simulink model "ev_project_1"  (R2024b)
settings: Solver=VariableStepAuto  StartTime=0.0  StopTime=20  RelTol=1e-3
libraries: spsIGBTDiodeLib x12, spsDiodeLib x6, spsSeriesRLCBranchLib x3, spsVoltageMeasurementLib x3, spsDCVoltageSourceLib x1, spsGroundLib x1, spsPermanentMagnetSynchronousMachineLib x1, spsThreePhaseVIMeasurementLib x1, sps_lib x1
settings Model: Creator=ravit  LastModifiedBy=ravit

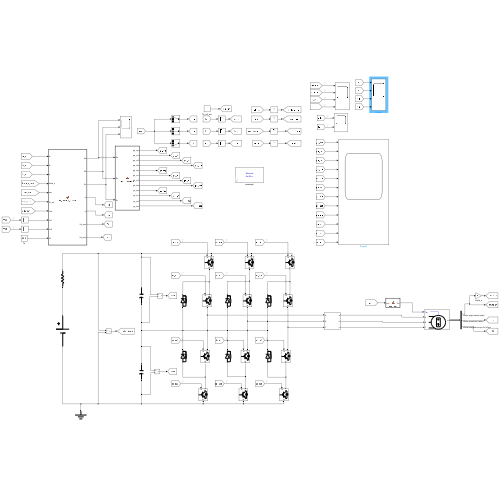
[thumbnail: Simulink's stored preview of the top-level diagram]
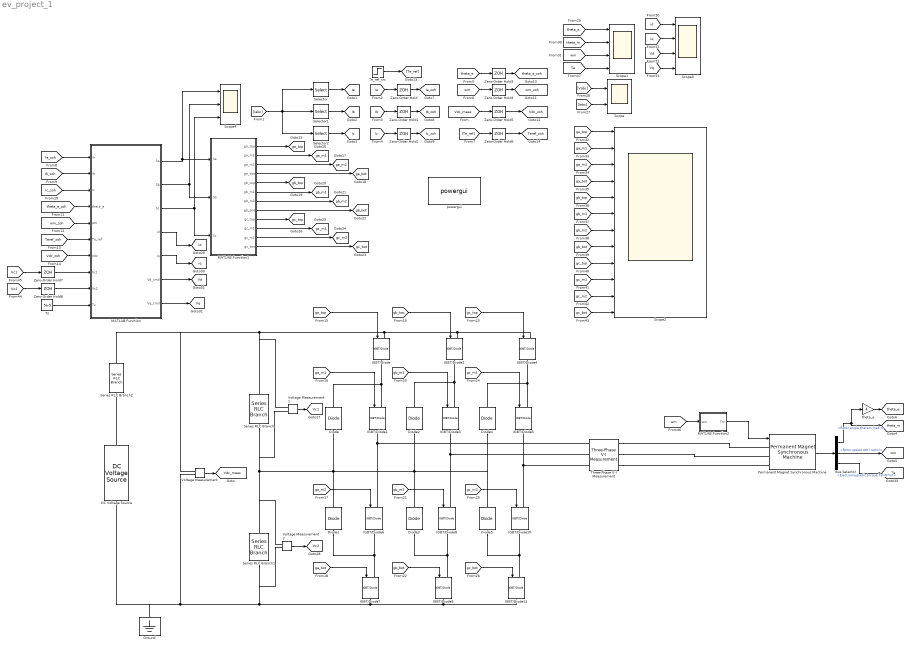
== system ev_project_1 ==
  Bus Selector : BusSelector  OutputSignals=Rotor angle thetam (rad),Rotor speed wm (rad/s),Electromagnetic torque Te (N*m)
  DC Voltage Source : spsDCVoltageSourceLib/DC Voltage Source  Amplitude=400  Measurements=None
  Diode{,1..5} (6 alike) : spsDiodeLib/Diode  Ron=0.001  Lon=0  Vf=0.8  IC=0  UseSnubber=0  Rs=500  Cs=250e-9  Measurements=off
  Ground : spsGroundLib/Ground  LConnTagsString=a
  IGBT/Diode{,1..11} (12 alike) : spsIGBTDiodeLib/IGBT//Diode  Ron=1e-3  Rs=1e5  Cs=inf  Measurements=off
  MATLAB Function : MATLAB Function  TreatAsAtomicUnit=on
  MATLAB Function1 : MATLAB Function  TreatAsAtomicUnit=on
  MATLAB Function2 : MATLAB Function  TreatAsAtomicUnit=on
  Permanent Magnet Synchronous Machine : spsPermanentMagnetSynchronousMachineLib/Permanent Magnet Synchronous Machine  NbPhases=3  FluxDistribution=Sinusoidal  RotorType=Salient-pole  MechanicalLoad=Torque Tm  PresetModel=No  ShowDetailedParameters=on  MeasurementBus=off  Resistance=0.05  Inductance=8.5e-3  dqInductances=[0.0005, 0.0011]  La=0.000395  MachineConstant=Flux linkage established by magnets (V.s)  Flux=0.045  VoltageCst=32.6484  TorqueCst=0.27  Flat=120  Mechanical=[0.01, 0.0004924, 4, 0]  PolePairs=4  InitialConditions=[0,0, 0,0]  InitialConditions5ph=[0 0 0 0 0 0]  RefAngle=90 degrees behind phase A axis (modified Park)  IterativeDiscreteModel=Trapezoidal non iterative  TsBlock=-1  TsPowergui=0
  Scope : Scope  NumInputPorts=2
  Scope1 : Scope  NumInputPorts=4
  Scope2 : Scope  NumInputPorts=12
  Scope3 : Scope  NumInputPorts=4
  Scope4 : Scope  NumInputPorts=3
  Selector : Selector  InputPortWidth=3  IndexOptions=Index vector (dialog)  Indices=[1]  OutputSizes=1
  Selector1 : Selector  InputPortWidth=3  IndexOptions=Index vector (dialog)  Indices=[2]  OutputSizes=1
  Selector2 : Selector  InputPortWidth=3  IndexOptions=Index vector (dialog)  Indices=[3]  OutputSizes=1
  Series RLC Branch : spsSeriesRLCBranchLib/Series RLC Branch  LConnTagsString=__new0  RConnTagsString=__new0  BranchType=C  Resistance=1  Inductance=1e-3  SetiL0=off  InitialCurrent=0  Capacitance=2200e-6  Setx0=on  InitialVoltage=200  Measurements=None
  Series RLC Branch1 : spsSeriesRLCBranchLib/Series RLC Branch  LConnTagsString=__new0  RConnTagsString=__new0  BranchType=C  Resistance=1  Inductance=1e-3  SetiL0=off  InitialCurrent=0  Capacitance=2200e-6  Setx0=on  InitialVoltage=200  Measurements=None
  Series RLC Branch2 : spsSeriesRLCBranchLib/Series RLC Branch  LConnTagsString=__new0  RConnTagsString=__new0  BranchType=R  Resistance=0.01  Inductance=1e-3  SetiL0=off  InitialCurrent=0  Capacitance=1e-6  Setx0=off  InitialVoltage=0  Measurements=None
  Te_ref_src : Step  Time=5  After=20  SampleTime=0
  Three-Phase V-I Measurement : spsThreePhaseVIMeasurementLib/Three-Phase V-I Measurement  VoltageMeasurement=phase-to-ground  SetLabelV=on  LabelV=Vabc  Vpu=off  VpuLL=off  CurrentMeasurement=yes  SetLabelI=on  LabelI=Iabc  Ipu=off  Pbase=100e6  Vbase=500e3  OutputType=Complex  PhasorSimulation=off  PSBequivalent=0
  Ts : Constant  Value=5e-5
  Voltage Measurement : spsVoltageMeasurementLib/Voltage Measurement  PhasorSimulation=off  OutputType=Complex  PSBequivalent=0
  Voltage Measurement1 : spsVoltageMeasurementLib/Voltage Measurement  PhasorSimulation=off  OutputType=Complex  PSBequivalent=0
  Voltage Measurement2 : spsVoltageMeasurementLib/Voltage Measurement  PhasorSimulation=off  OutputType=Complex  PSBequivalent=0
  Zero-Order Hold{,1..8} (9 alike) : ZeroOrderHold  SampleTime=5e-5
  powergui : sps_lib/powergui  Priority=1  SimulationMode=Discrete  SampleTime=50e-6  frequency=60  Iterations=50  frequencyindice=0  Pbase=100e6  ErrMax=1e-4  UnitsV=kV  UnitsW=MW  buscounter=0  FunctionMessages=off  echomessages=off  EnableUseOfTLC=off  CurrentSourceSwitches=off  DisableSnubberDevices=off  DisableRonSwitches=off  DisableVfSwitches=off  DisplayEquations=off  AutomaticDiscreteSolvers=off  SolverType=Tustin/Backward Euler (TBE)  Interpol=off  ExternalGateDelay=off  methode=off  Ts=100  x0status=blocks  SPID=on  SwTol=0  HookPort=off  NonlinearTolerance=1e-4  nMaxIteration=100  ContinueOnMaxIteration=off  RestoreLinks=warning  ResistiveCurrentMeasurement=off  Frange=[0:2:500]  Ylog=off  Xlog=on  ShowGrid=off  save=off  variable=ZData  structure=0  ZoomFFT=off  StartTime=0.0  cycles=1  DisplayStyle=1  fundamental=60  FreqAxis=off  MaxFrequency=1000  frequencyindicesteady=1  RmsSteady=1  display=off
  theta_e : Gain  Gain=4
  tag scope: Ia=global, Ia_zoh=global, Ib=global, Ib_zoh=global, Ic=global, Ic_zoh=global, Te=global, Teref_zoh=global, Vc1=global, Vc2=global, Vd=global, Vdc_meas=global, Vdc_zoh=global, Vq=global, ga_bot=global, ga_m1=global, ga_m2=global, ga_top=global, gb_bot=global, gb_m1=global, gb_m2=global, gb_top=global, gc_bot=global, gc_m1=global, gc_m2=global, gc_top=global, id=global, iq=global, theta_e=global, theta_e_zoh=global, theta_m=global, wm=global, wm_zoh=global
  wires:
  Voltage Measurement/1 -> [Vdc_meas]
  Permanent Magnet Synchronous Machine/1 -> Bus Selector/1
  [Iabc] -> Selector2/1, Selector/1, Selector1/1
  Selector/1 -> [Ia]
  Selector1/1 -> [Ib]
  Selector2/1 -> [Ic]
  Bus Selector/1 -> [theta_m], theta_e/1  "<Rotor angle thetam (rad)>"
  Bus Selector/2 -> [wm]  "<Rotor speed wm (rad/s)>"
  theta_e/1 -> [theta_e]
  [Ia] -> Zero-Order Hold/1
  [Ib] -> Zero-Order Hold1/1
  [Ic] -> Zero-Order Hold2/1
  Zero-Order Hold/1 -> [Ia_zoh]
  Zero-Order Hold1/1 -> [Ib_zoh]
  Zero-Order Hold2/1 -> [Ic_zoh]
  [theta_e] -> Zero-Order Hold3/1
  Zero-Order Hold3/1 -> [theta_e_zoh]
  [wm] -> Zero-Order Hold4/1
  Zero-Order Hold4/1 -> [wm_zoh]
  [Vdc_meas] -> Zero-Order Hold5/1
  Zero-Order Hold5/1 -> [Vdc_zoh]
  Te_ref_src/1 -> [Te_ref]
  [Te_ref] -> Zero-Order Hold6/1
  Zero-Order Hold6/1 -> [Teref_zoh]
  [Ia_zoh] -> MATLAB Function/1(ia)
  [Ib_zoh] -> MATLAB Function/2(ib)
  [Ic_zoh] -> MATLAB Function/3(ic)
  [theta_e_zoh] -> MATLAB Function/4(theta_e)
  [wm_zoh] -> MATLAB Function/5(wm)
  [Teref_zoh] -> MATLAB Function/6(Te_ref)
  [Vdc_zoh] -> MATLAB Function/7(Vdc)
  Ts/1 -> MATLAB Function/10(Ts)
  MATLAB Function/1(Sa) -> Scope4/1, MATLAB Function1/1(Sa)
  MATLAB Function/2(Sb) -> MATLAB Function1/2(Sb), Scope4/2
  MATLAB Function/3(Sc) -> MATLAB Function1/3(Sc), Scope4/3
  MATLAB Function1/1(ga_top) -> [ga_top]
  MATLAB Function1/2(ga_m1) -> [ga_m1]
  MATLAB Function1/3(ga_m2) -> [ga_m2]
  MATLAB Function1/4(ga_bot) -> [ga_bot]
  MATLAB Function1/5(gb_top) -> [gb_top]
  MATLAB Function1/6(gb_m1) -> [gb_m1]
  MATLAB Function1/7(gb_m2) -> [gb_m2]
  MATLAB Function1/8(gb_bot) -> [gb_bot]
  MATLAB Function1/12(gc_bot) -> [gc_bot]
  MATLAB Function1/11(gc_m2) -> [gc_m2]
  MATLAB Function1/10(gc_m1) -> [gc_m1]
  MATLAB Function1/9(gc_top) -> [gc_top]
  [ga_top] -> IGBT/Diode/1
  [ga_m1] -> IGBT/Diode1/1
  [ga_m2] -> IGBT/Diode6/1
  [ga_bot] -> IGBT/Diode7/1
  [gb_top] -> IGBT/Diode2/1
  [gb_m1] -> IGBT/Diode3/1
  [gb_m2] -> IGBT/Diode8/1
  [gb_bot] -> IGBT/Diode9/1
  [gc_top] -> IGBT/Diode4/1
  [gc_m2] -> IGBT/Diode10/1
  [gc_m1] -> IGBT/Diode5/1
  [gc_bot] -> IGBT/Diode11/1
  [Iabc] -> Scope/2
  [Vabc] -> Scope/1
  [theta_e] -> Scope1/1
  [theta_m] -> Scope1/2
  [wm] -> Scope1/3
  [ga_top] -> Scope2/1
  [ga_m1] -> Scope2/2
  [ga_m2] -> Scope2/3
  [ga_bot] -> Scope2/4
  [gb_top] -> Scope2/5
  [gb_m1] -> Scope2/6
  [gb_m2] -> Scope2/7
  [gb_bot] -> Scope2/8
  [gc_top] -> Scope2/9
  [gc_m1] -> Scope2/10
  [gc_m2] -> Scope2/11
  [gc_bot] -> Scope2/12
  Voltage Measurement1/1 -> [Vc1]
  Voltage Measurement2/1 -> [Vc2]
  [Vc1] -> Zero-Order Hold7/1
  [Vc2] -> Zero-Order Hold8/1
  Zero-Order Hold7/1 -> MATLAB Function/8(Vc1)
  Zero-Order Hold8/1 -> MATLAB Function/9(Vc2)
  [wm] -> MATLAB Function2/1(wm)
  MATLAB Function2/1(Tm) -> Permanent Magnet Synchronous Machine/1
  MATLAB Function/4(id) -> [id]
  MATLAB Function/5(iq) -> [iq]
  MATLAB Function/6(Vd_cmd) -> [Vd]
  MATLAB Function/7(Vq_cmd) -> [Vq]
  [id] -> Scope3/1
  [iq] -> Scope3/2
  [Vd] -> Scope3/3
  [Vq] -> Scope3/4
  Bus Selector/3 -> [Te]  "<Electromagnetic torque Te (N*m)>"
  [Te] -> Scope1/4
  connections:
  IGBT/Diode5/LConn1 -- Diode4/RConn1 -- IGBT/Diode4/RConn1
  IGBT/Diode3/LConn1 -- Diode2/RConn1 -- IGBT/Diode2/RConn1
  IGBT/Diode1/LConn1 -- Diode/RConn1 -- IGBT/Diode/RConn1
  IGBT/Diode/LConn1 -- Voltage Measurement1/LConn1 -- Series RLC Branch/LConn1 -- Series RLC Branch2/LConn1 -- Voltage Measurement/LConn1 -- IGBT/Diode4/LConn1 -- IGBT/Diode2/LConn1
  IGBT/Diode7/LConn1 -- Diode1/LConn1 -- IGBT/Diode6/RConn1
  IGBT/Diode11/LConn1 -- IGBT/Diode10/RConn1 -- Diode5/LConn1
  IGBT/Diode9/LConn1 -- Diode3/LConn1 -- IGBT/Diode8/RConn1
  IGBT/Diode7/RConn1 -- Series RLC Branch1/RConn1 -- Voltage Measurement2/LConn2 -- DC Voltage Source/LConn1 -- Ground/LConn1 -- Voltage Measurement/LConn2 -- IGBT/Diode11/RConn1 -- IGBT/Diode9/RConn1
  Diode1/RConn1 -- Diode/LConn1 -- Series RLC Branch/RConn1 -- Voltage Measurement1/LConn2 -- Series RLC Branch1/LConn1 -- Voltage Measurement2/LConn1 -- Diode5/RConn1 -- Diode4/LConn1 -- Diode3/RConn1 -- Diode2/LConn1
  IGBT/Diode8/LConn1 -- Three-Phase V-I Measurement/LConn2 -- IGBT/Diode3/RConn1
  IGBT/Diode10/LConn1 -- Three-Phase V-I Measurement/LConn3 -- IGBT/Diode5/RConn1
  IGBT/Diode6/LConn1 -- Three-Phase V-I Measurement/LConn1 -- IGBT/Diode1/RConn1
  DC Voltage Source/RConn1 -- Series RLC Branch2/RConn1
  Three-Phase V-I Measurement/RConn1 -- Permanent Magnet Synchronous Machine/LConn1
  Three-Phase V-I Measurement/RConn2 -- Permanent Magnet Synchronous Machine/LConn2
  Three-Phase V-I Measurement/RConn3 -- Permanent Magnet Synchronous Machine/LConn3

== matlab function ev_project_1/MATLAB Function1 ==
  data: Sa input; ga_top output; Sb input; Sc input; ga_m1 output; ga_m2 output; ga_bot output; gb_top output; gb_m1 output; gb_m2 output; gb_bot output; gc_top output; gc_m1 output; gc_m2 output; gc_bot output
function [ga_top,ga_m1,ga_m2,ga_bot, gb_top,gb_m1,gb_m2,gb_bot, gc_top,gc_m1,gc_m2,gc_bot] = gate_decoder(Sa, Sb, Sc)
%#codegen
% Decodes each leg's 3-level state (-1, 0, +1) into 4 physical gate
% signals for a diode-clamped (NPC) leg: top main switch, two inner
% (clamp-adjacent) switches, bottom main switch.
%
% NPC switching table (per leg):
%   State +1 (P): S1=ON, S2=ON,  S3=OFF, S4=OFF
%   State  0 (O): S1=OFF,S2=ON,  S3=ON,  S4=OFF
%   State -1 (N): S1=OFF,S2=OFF, S3=ON,  S4=ON
% Note: each inner switch spans TWO adjacent states, not one.

[ga_top, ga_m1, ga_m2, ga_bot] = leg_decode(Sa);
[gb_top, gb_m1, gb_m2, gb_bot] = leg_decode(Sb);
[gc_top, gc_m1, gc_m2, gc_bot] = leg_decode(Sc);

end

function [g_top, g_m1, g_m2, g_bot] = leg_decode(S)
  g_top = double(S == 1);
  g_m1  = double(S == 1 | S == 0);   % ON for P and O
  g_m2  = double(S == 0 | S == -1);  % ON for O and N
  g_bot = double(S == -1);
end

== matlab function ev_project_1/MATLAB Function ==
  data: ia input; Sa output; ib input; ic input; theta_e input; wm input; Te_ref input; Vdc input; Vc1 input; Vc2 input; Ts input; Sb output; Sc output; id output; iq output; Vd_cmd output; Vq_cmd output
function [Sa, Sb, Sc, id, iq, Vd_cmd, Vq_cmd] = pir_current_control(ia, ib, ic, theta_e, wm, Te_ref, Vdc, Vc1, Vc2, Ts)
%#codegen
% PIR (PI + Resonant) dq current control for 3-level NPC PMSM drive.
% Replaces FCS-MPTC. Outputs Sa,Sb,Sc feed the existing gate_decoder chart
% unchanged (same -1/0/+1 leg-level convention).

% --- Machine parameters (must match PMSM block mask) ---
Rs        = 0.05;
Ld        = 0.50e-3;
Lq        = 1.10e-3;
lambda_pm = 0.045;
P         = 4;

% --- Current-loop PI gains (pole-zero cancellation, ~1 kHz bandwidth) ---
% Kp = L*wc, Ki = Rs*wc.  RE-TUNE if you change bandwidth or parameters.
wc_i = 2*pi*1000;
Kp_d = Ld*wc_i;   Ki_d = Rs*wc_i;
Kp_q = Lq*wc_i;   Ki_q = Rs*wc_i;

% --- Resonant gains, tuned at 6*we. Start near Kp, then tune from FFT results ---
Kr_d = Kp_d;
Kr_q = Kp_q;

% --- Neutral-point balance PI (slow, low bandwidth) ---
Kp_np = 0.01;
Ki_np = 1.0;

% --- Reference-frame offset: PMSM mask uses "90 deg behind phase A"
%     (modified Park). Flip the sign here if the Phase-1 open-loop
%     θ-convention test showed the opposite offset is correct. ---
THETA_OFFSET = pi/2;

% --- Persistent controller/observer states ---
persistent id_int iq_int x1d x2d x1q x2q np_int init
if isempty(init)
    id_int = 0; iq_int = 0;
    x1d = 0; x2d = 0; x1q = 0; x2q = 0;
    np_int = 0;
    init = true;
end

% --- Corrected angle, Clarke/Park ---
theta_use = theta_e + THETA_OFFSET;
ialpha = ia;
ibeta  = (ia + 2*ib) / sqrt(3);
id = ialpha*cos(theta_use) + ibeta*sin(theta_use);
iq = -ialpha*sin(theta_use) + ibeta*cos(theta_use);

we = P*wm;

% --- Current references (Id*=0, MTPA can replace this later) ---
id_ref = 0;
iq_ref = Te_ref / (1.5*P*lambda_pm);

ed = id_ref - id;
eq = iq_ref - iq;

% --- PI (forward Euler, with anti-windup clamp) ---
id_int = id_int + Ki_d*ed*Ts;
iq_int = iq_int + Ki_q*eq*Ts;
id_int = max(min(id_int, Vdc/2), -Vdc/2);
iq_int = max(min(iq_int, Vdc/2), -Vdc/2);

% --- Resonant term at wr = 6*we, symplectic Euler with pre-warped wr ---
% Pre-warping keeps the resonant peak accurate even at high wr*Ts.
wr = 6*we;
if wr > 1e-3
    wr_dig = (2/Ts)*tan(min(wr*Ts/2, 1.55));  % clamp guards against tan blow-up
else
    wr_dig = 0;
end

x2d = x2d + Ts*(-wr_dig^2*x1d + ed);
x1d = x1d + Ts*x2d;
res_d = Kr_d*x2d;

x2q = x2q + Ts*(-wr_dig^2*x1q + eq);
x1q = x1q + Ts*x2q;
res_q = Kr_q*x2q;

% --- Combine PI + Resonant + decoupling feedforward ---
Vd_cmd = Kp_d*ed + id_int + res_d - we*Lq*iq;
Vq_cmd = Kp_q*eq + iq_int + res_q + we*Ld*id + we*lambda_pm;

% --- Neutral-point balance: PI on Vc1-Vc2, injected as common-mode offset ---
dVc = Vc1 - Vc2;
np_int = np_int + dVc*Ts;
v0 = Kp_np*dVc + Ki_np*np_int;

% --- Inverse Park/Clarke ---
Valpha = Vd_cmd*cos(theta_use) - Vq_cmd*sin(theta_use);
Vbeta  = Vd_cmd*sin(theta_use) + Vq_cmd*cos(theta_use);

Va = Valpha            + v0;
Vb = -0.5*Valpha + (sqrt(3)/2)*Vbeta + v0;
Vc = -0.5*Valpha - (sqrt(3)/2)*Vbeta + v0;

% --- Normalize to modulation index, then Nearest-Level Modulation ---
ma = max(min(Va/(Vdc/2), 1), -1);
mb = max(min(Vb/(Vdc/2), 1), -1);
mc = max(min(Vc/(Vdc/2), 1), -1);

Sa = round(ma);
Sb = round(mb);
Sc = round(mc);

end

== matlab function ev_project_1/MATLAB Function2 ==
  data: wm input; Tm output
function Tm = road_load(wm)
%#codegen
% Speed-feedback mechanical load: rolling resistance + viscous + aero drag.
% Acts as a virtual dynamometer so wm settles to a stable equilibrium
% instead of the near-integrator behavior of PMSM friction alone.

Tc = 4;         % Nm, rolling resistance / static friction
B  = 0.02;      % N.m.s, linear viscous loss
K  = 1.111e-4;  % N.m.s^2, aerodynamic drag

% Smooth sign to avoid a hard discontinuity at wm=0 on a discrete solver
% (a true sign() can chatter right at standstill).
eps_w = 0.5;   % rad/s, smoothing width -- small relative to wm_rated
sign_smooth = tanh(wm/eps_w);

Tm = Tc*sign_smooth + B*wm + K*wm*abs(wm);

end
